simulink model "Assertion1"  (R2017b)
settings: Solver=FixedStepDiscrete  StartTime=0.0  StopTime=10.0  FixedStep=0.200000  RelTol=1e-3
libraries: simulink x1
settings Model: Creator=hbourbou  LastModifiedBy=hbourbou
settings OptimizationCC: LifeSpan=inf
settings DebuggingCC: SFExecutionAtInitializationDiag=none
settings HardwareCC: ProdBitPerSizeT=32  ProdBitPerPtrDiffT=32  ProdWordSize=32  ProdHWDeviceType=Specified
settings CodeAppCC: StateflowObjectComments=on

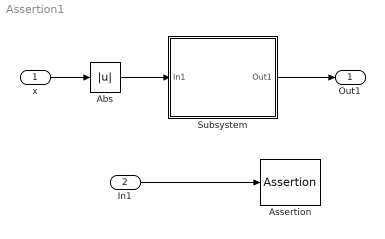
== system Assertion1 ==
  x : Inport
  In1 : Inport  Port=2  PortDimensions=3
  Abs : Abs
  Assertion : Assertion  StopWhenAssertionFail=off
  Subsystem : Subsystem  TreatAsAtomicUnit=on
  Out1 : Outport
  wires:
  x/1 -> Abs/1
  Subsystem/1(Out1) -> Out1/1
  Abs/1 -> Subsystem/1(In1)
  In1/1 -> Assertion/1

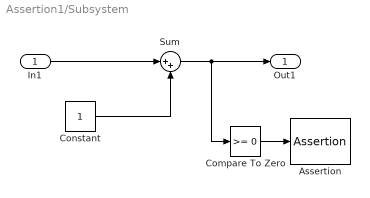
== system Assertion1/Subsystem ==
  In1 : Inport
  Assertion : Assertion  StopWhenAssertionFail=off
  Compare To Zero : simulink/Logic and Bit Operations/Compare To Zero  relop=>=  OutDataTypeStr=boolean
  Constant : Constant
  Sum : Sum  Inputs=|++
  Out1 : Outport
  wires:
  In1/1 -> Sum/1
  Constant/1 -> Sum/2
  Sum/1 -> Compare To Zero/1, Out1/1
  Compare To Zero/1 -> Assertion/1
